simulink model "QPSK"  (R2017a)
settings: Solver=VariableStepAuto  StartTime=0.0  StopTime=10.0  RelTol=1e-3
libraries: commutil2 x2, commchan3 x1, commrandsrc3 x1, dspsrcs4 x1, commsink2 x1, dspswit3 x1
settings Model: Creator=81228  LastModifiedBy=81228

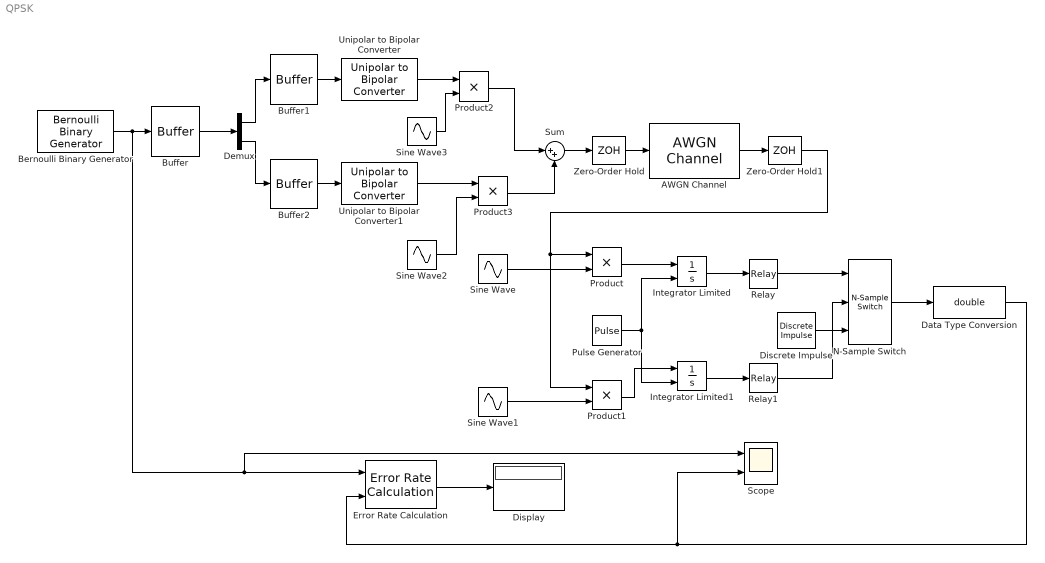
== system QPSK ==
  AWGN Channel : commchan3/AWGN Channel  InputProcessing=Columns as channels (frame based)  seed=67  noiseMode="Signal to noise ratio  (Eb/No)"  EbNodB=10  EsNodB=10  SNRdB=10  bitsPerSym=1  Ps=1  Tsym=1  variance=1
  Bernoulli Binary Generator : commrandsrc3/Bernoulli Binary Generator  ProbabilityOfZero=0.5  SeedSource=Auto  Seed=0  SampleTime=0.01  SamplesPerFrame=1  OutputDataType=double  SimulateUsing=Interpreted execution
  Buffer : Buffer  OutputFrames=off
  Buffer1 : Buffer  OutputFrames=off
  Buffer2 : Buffer  OutputFrames=off
  Data Type Conversion : DataTypeConversion  OutDataTypeStr=double
  Demux : Demux  Outputs=2
  Discrete Impulse : dspsrcs4/Discrete  Impulse  Delay=0  SampleTime=1  FrameSample=1  OutputFrames=off  dataType=double  isSigned=on  wordLen=16  udDataType=sfix(16)  fracBitsMode=Best precision  numFracBits=15  OutDataTypeStr=double  LastOutDataTypeStr=double
  Display : Display
  Error Rate Calculation : commsink2/Error Rate Calculation  N=0  st_delay=0  cp_mode=Entire frame  subframe=[]  PMode=Port  WsName=ErrorVec  RsMode2=off  stop=off  numErr=100  maxBits=1e6
  Integrator Limited : Integrator  InitialConditionSource=external  LimitOutput=on  UpperSaturationLimit=2  LowerSaturationLimit=0
  Integrator Limited1 : Integrator  InitialConditionSource=external  LimitOutput=on  UpperSaturationLimit=2  LowerSaturationLimit=0
  N-Sample Switch : dspswit3/N-Sample Switch  N=8  reset=on  TriggerType=Rising edge  Ts=0.1
      settings: SourceProductName=DSP System Toolbox  SourceProductBaseCode=DS
  Product{,1..3} (4 alike) : Product
  Pulse Generator : DiscretePulseGenerator  PulseType=Time based  Period=10  PulseWidth=5
  Relay : Relay
  Relay1 : Relay
  Scope : Scope  NumInputPorts=2
  Sine Wave{,1..3} (4 alike) : Sin  Frequency=100*pi  SampleTime=0.01
  Sum : Sum  Inputs=|++
  Unipolar to Bipolar Converter : commutil2/Unipolar to Bipolar Converter  M=4  polarity=Positive  dataType=Inherit via internal rule
      settings: SourceProductName=Communications System Toolbox
  Unipolar to Bipolar Converter1 : commutil2/Unipolar to Bipolar Converter  M=4  polarity=Positive  dataType=Inherit via internal rule
      settings: SourceProductName=Communications System Toolbox
  Zero-Order Hold : ZeroOrderHold  SampleTime=0.02
  Zero-Order Hold1 : ZeroOrderHold  SampleTime=0.02
  wires:
  Bernoulli Binary Generator/1 -> Error Rate Calculation/1, Scope/1, Buffer/1
  Buffer/1 -> Demux/1
  Demux/1 -> Buffer1/1
  Demux/2 -> Buffer2/1
  Buffer1/1 -> Unipolar to Bipolar Converter/1
  Buffer2/1 -> Unipolar to Bipolar Converter1/1
  Unipolar to Bipolar Converter/1 -> Product2/1
  Sine Wave3/1 -> Product2/2
  Product2/1 -> Sum/1
  Unipolar to Bipolar Converter1/1 -> Product3/1
  Product3/1 -> Sum/2
  Sine Wave2/1 -> Product3/2
  Sum/1 -> Zero-Order Hold/1
  Zero-Order Hold/1 -> AWGN Channel/1
  AWGN Channel/1 -> Zero-Order Hold1/1
  Sine Wave/1 -> Product/2
  Zero-Order Hold1/1 -> Product/1, Product1/1
  Sine Wave1/1 -> Product1/2
  Integrator Limited/1 -> Relay/1
  Product/1 -> Integrator Limited/1
  Pulse Generator/1 -> Integrator Limited1/2, Integrator Limited/2
  Product1/1 -> Integrator Limited1/1
  Integrator Limited1/1 -> Relay1/1
  Error Rate Calculation/1 -> Display/1
  Data Type Conversion/1 -> Scope/2, Error Rate Calculation/2
  Discrete Impulse/1 -> N-Sample Switch/3
  Relay/1 -> N-Sample Switch/1
  N-Sample Switch/1 -> Data Type Conversion/1
  Relay1/1 -> N-Sample Switch/2
